simulink model "SkidSteeringControl"  (Simulink 8.9)
settings: Solver=VariableStepAuto  StartTime=0.0  StopTime=100  MaxStep=0.01  RelTol=1e-3
PreLoadFcn:
  | % Vehicle parameters
  | m = 1000;  % Vehicle mass
  | fR = 0.3;  % Front wheel radius
  | rR = 0.3;  % Rear wheel radius
  | J_front = 0.5;  % Front wheel moment of inertia
  | J_rear = 0.5;  % Rear wheel moment of inertia
  | J_engine = 0.01; % Engine moment of inertia
  | trans_ratio = 2.0;  % Transmission gear ratio
  | drive_ratio = 2.0;  % Final drive gear ratio
  | h = 0.5;   % Vehicle CG height above ground
  | 
  | % Aerodynamic load
  | cw = 0.34;  % Drag coefficient
  | rho = 1.18; % Air density
  | A_f = 1;    % Frontal area
  | 
  | 
  | %tire parameters
  | radiusWheel = 16*2.54/100;
  | inertiaLateral = 25*(radiusWheel)^2;
  | tireStiffness = 200000;
  | tireDamping = 1000;
StopFcn:
  | %%
  | close all;
  | figure;plot(disp_x,disp_y);grid on;axis('tight');
  | title('Vehicle Displacement Plot');
  | xlabel('Displacement X(m)');ylabel('Displacement Y(m)');
  | %%
  | figure;
  | subplot(2,1,1);
  | plot(desired_speedFL.time, desired_speedFL.signals.values,'g');grid on;hold on;
  | plot(desired_speedFR.time, desired_speedFR.signals.values,'b');grid on;
  | title('Desired Wheel Speed');
  | legend('Wheel Speed FL','Wheel Speed FR');
  | subplot(2,1,2);
  | plot(ref_speedFL.time, ref_speedFL.signals.values,'g');grid on;hold on;
  | plot(ref_speedFR.time, ref_speedFR.signals.values,'b');grid on;
  | title('Reference Wheel Speed(Slip Compensated)');
  | legend('Wheel Speed FL','Wheel Speed FR');
  | %%
  | figure;plot(yaw_rate.time,yaw_rate.signals.values);grid on;
  | title('Vehicle Yaw Rate');
  | xlabel('time(s)');ylabel('Yaw Rate(rad/s)');
  | %%
  | figure;
  | subplot(2,1,1);
  | plot(slip_WheelFL.time, slip_WheelFL.signals.values);grid on;
  | title('Wheel Slip Front Left');
  | xlabel('time(s)');ylabel('Slip Ratio');
  | subplot(2,1,2);
  | plot(slip_WheelFR.time, slip_WheelFR.signals.values);grid on;
  | title('Wheel Slip Front Right');
  | xlabel('time(s)');ylabel('Slip Ratio');
  | %%
  | figure;
  | subplot(2,1,1);
  | plot(torque_WheelFL.time, torque_WheelFL.signals.values);grid on;
  | title('Wheel Torque Front Left');
  | xlabel('time(s)');ylabel('Torque(Nm)');
  | subplot(2,1,2);
  | plot(torque_WheelFR.time, torque_WheelFR.signals.values);grid on;
  | title('Wheel Torque Front Right');
  | xlabel('time(s)');ylabel('Torque(Nm)');
libraries: nesl_utility x8, fl_lib x4, sdl_lib x4, simulink_extras x2, simulink x1
(part 1 of 2)
settings Model: Creator=divye  LastModifiedBy=divye
settings DataIOCC: LimitDataPoints=off  SaveFormat=Dataset  SignalLoggingSaveFormat=Dataset
settings OptimizationCC: LifeSpan=auto
settings DebuggingCC: UnderspecifiedInitializationDetection=Simplified  MergeDetectMultiDrivingBlocksExec=error  FcnCallInpInsideContextMsg=error  StateNameClashWarn=none  SFUnexpectedBacktrackingDiag=error  SFNoUnconditionalDefaultTransitionDiag=error  SFExecutionAtInitializationDiag=warning
settings HardwareCC: ProdBitPerPointer=64  ProdBitPerSizeT=64  ProdBitPerPtrDiffT=64  ProdLargestAtomicFloat=Float  ProdIntDivRoundTo=Zero  ProdEndianess=LittleEndian  ProdWordSize=64  ProdHWDeviceType=Intel->x86-64 (Windows64)
settings ModelReferenceCC: PropagateSignalLabelsOutOfModel=on
settings GRTTargetCC: TargetLangStandard=C99 (ISO)  GeneratePreprocessorConditionals=Use local settings  CombineOutputUpdateFcns=on  GRTInterface=off
settings ConfigComp: CovMetricSettings=dwe  CovHtmlReporting=off  CovSaveCumulativeToWorkspaceVar=off  CovSaveSingleToWorkspaceVar=off  CovExternalEMLEnable=on

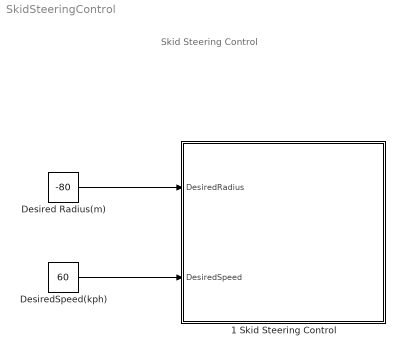
== system SkidSteeringControl ==
  note: Skid Steering Control
  1 Skid Steering Control : Subsystem
  Desired Radius(m) : Constant  Value=-80
  DesiredSpeed(kph) : Constant  Value=60
  wires:
  Desired Radius(m)/1 -> 1 Skid Steering Control/1(DesiredRadius)
  DesiredSpeed(kph)/1 -> 1 Skid Steering Control/2(DesiredSpeed)

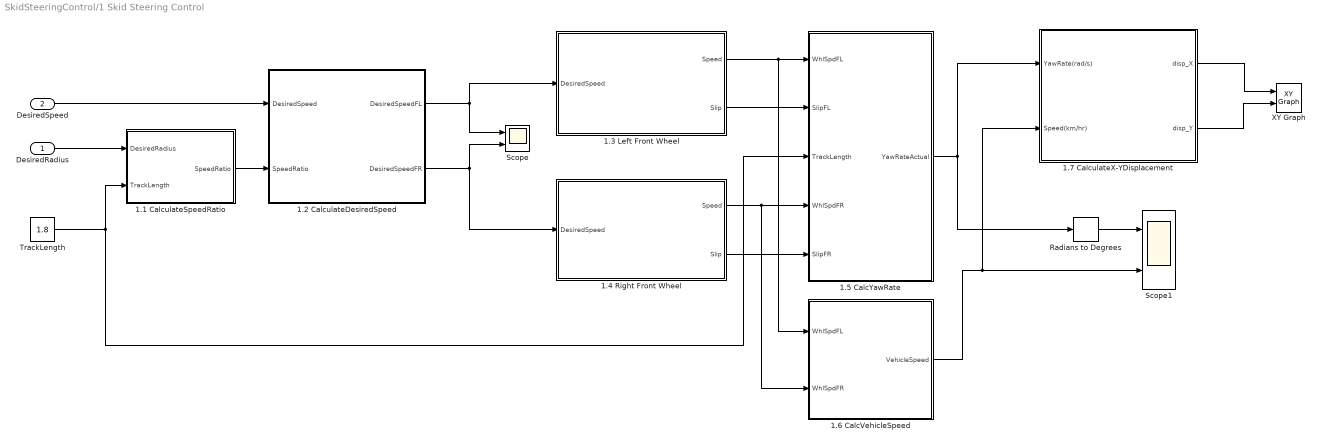
== system SkidSteeringControl/1 Skid Steering Control ==
  DesiredRadius : Inport
  DesiredSpeed : Inport  Port=2
  1.1 CalculateSpeedRatio : Subsystem
  1.2 CalculateDesiredSpeed : Subsystem
  1.3 Left Front Wheel : Subsystem
  1.4 Right Front Wheel : Subsystem
  1.5 CalcYawRate : Subsystem
  1.6 CalcVehicleSpeed : Subsystem
  1.7 CalculateX-YDisplacement : Subsystem
  Radians to Degrees : simulink_extras/Transformations/Radians to Degrees
  Scope : Scope  NumInputPorts=2
  Scope1 : Scope  NumInputPorts=2
  TrackLength : Constant  Value=1.8
  XY Graph : simulink/Sinks/XY Graph  xmin=-200  xmax=200  ymin=-200  ymax=200  st=-1
  wires:
  1.3 Left Front Wheel/1(Speed) -> 1.5 CalcYawRate/1(WhlSpdFL), 1.6 CalcVehicleSpeed/1(WhlSpdFL)
  TrackLength/1 -> 1.5 CalcYawRate/3(TrackLength), 1.1 CalculateSpeedRatio/2(TrackLength)
  1.5 CalcYawRate/1(YawRateActual) -> Radians to Degrees/1, 1.7 CalculateX-YDisplacement/1(YawRate(rad/s))
  1.6 CalcVehicleSpeed/1(VehicleSpeed) -> Scope1/2, 1.7 CalculateX-YDisplacement/2(Speed(km/hr))
  1.4 Right Front Wheel/1(Speed) -> 1.5 CalcYawRate/4(WhlSpdFR), 1.6 CalcVehicleSpeed/2(WhlSpdFR)
  1.4 Right Front Wheel/2(Slip) -> 1.5 CalcYawRate/5(SlipFR)
  1.3 Left Front Wheel/2(Slip) -> 1.5 CalcYawRate/2(SlipFL)
  DesiredSpeed/1 -> 1.2 CalculateDesiredSpeed/1(DesiredSpeed)
  Radians to Degrees/1 -> Scope1/1
  1.7 CalculateX-YDisplacement/1(disp_X) -> XY Graph/1
  1.7 CalculateX-YDisplacement/2(disp_Y) -> XY Graph/2
  1.2 CalculateDesiredSpeed/2(DesiredSpeedFR) -> 1.4 Right Front Wheel/1(DesiredSpeed), Scope/2
  1.2 CalculateDesiredSpeed/1(DesiredSpeedFL) -> Scope/1, 1.3 Left Front Wheel/1(DesiredSpeed)
  DesiredRadius/1 -> 1.1 CalculateSpeedRatio/1(DesiredRadius)
  1.1 CalculateSpeedRatio/1(SpeedRatio) -> 1.2 CalculateDesiredSpeed/2(SpeedRatio)

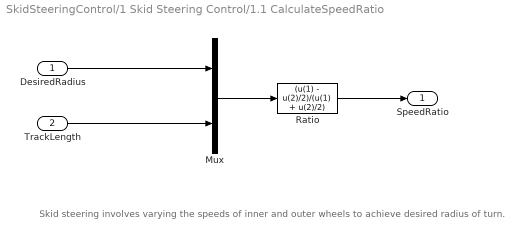
== system SkidSteeringControl/1 Skid Steering Control/1.1 CalculateSpeedRatio ==
  note: Skid steering involves varying the speeds of inner and outer wheels to achieve desired radius of turn.
  DesiredRadius : Inport
  TrackLength : Inport  Port=2
  Mux : Mux  Inputs=2
  Ratio : Fcn  Expr=(u(1) - u(2)/2)/(u(1) + u(2)/2)
  SpeedRatio : Outport
  wires:
  Ratio/1 -> SpeedRatio/1
  DesiredRadius/1 -> Mux/1
  Mux/1 -> Ratio/1
  TrackLength/1 -> Mux/2

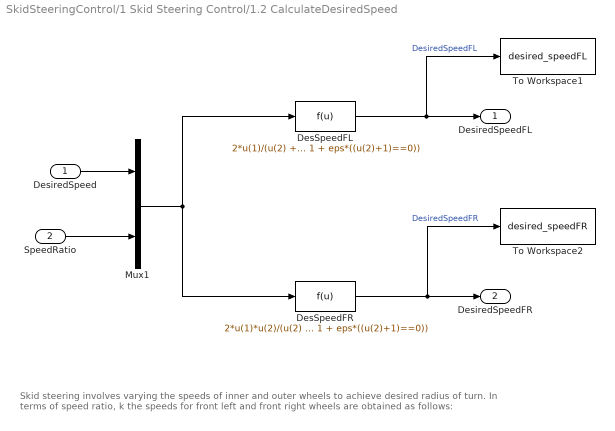
== system SkidSteeringControl/1 Skid Steering Control/1.2 CalculateDesiredSpeed ==
  note: Skid steering involves varying the speeds of inner and outer wheels to achieve desired radius of turn.
      |
      | In terms of speed ratio, k the speeds for front left and front right wheels are obtained as follows:
  DesiredSpeed : Inport
  SpeedRatio : Inport  Port=2
  DesSpeedFL : Fcn  Expr=2*u(1)/(u(2) + 1 + eps*((u(2)+1)==0))
  DesSpeedFR : Fcn  Expr=2*u(1)*u(2)/(u(2) + 1 + eps*((u(2)+1)==0))
  Mux1 : Mux  Inputs=2
  To Workspace1 : ToWorkspace  VariableName=desired_speedFL  SaveFormat=Structure With Time  SampleTime=-1
  To Workspace2 : ToWorkspace  VariableName=desired_speedFR  SaveFormat=Structure With Time  SampleTime=-1
  DesiredSpeedFL : Outport
  DesiredSpeedFR : Outport  Port=2
  wires:
  Mux1/1 -> DesSpeedFL/1, DesSpeedFR/1
  DesSpeedFR/1 -> To Workspace2/1, DesiredSpeedFR/1  "DesiredSpeedFR"
  DesSpeedFL/1 -> To Workspace1/1, DesiredSpeedFL/1  "DesiredSpeedFL"
  DesiredSpeed/1 -> Mux1/1
  SpeedRatio/1 -> Mux1/2

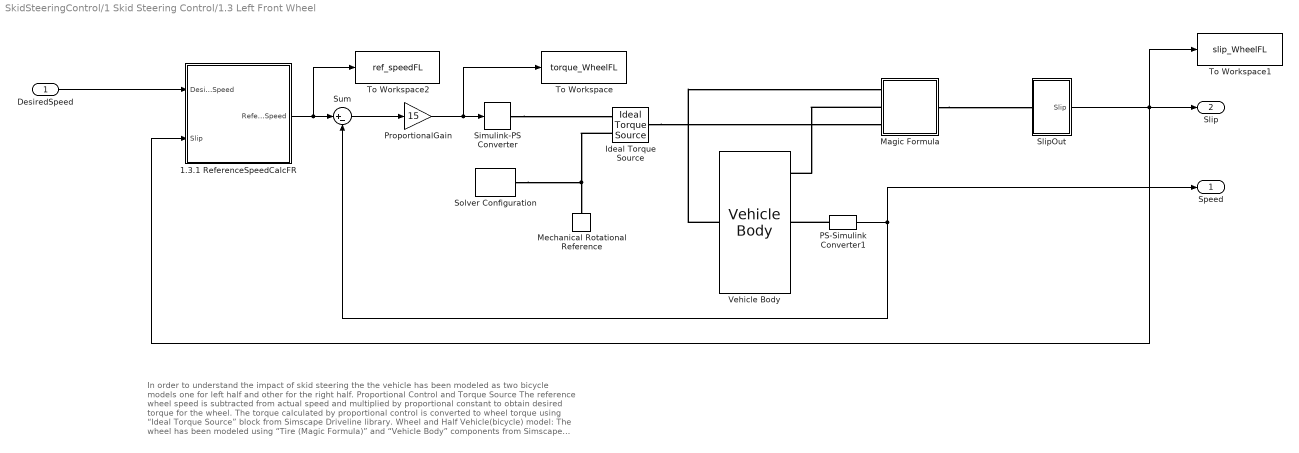
== system SkidSteeringControl/1 Skid Steering Control/1.3 Left Front Wheel ==
  note: In order to understand the impact of skid steering the the vehicle has been modeled as two bicycle models one for left half and other for the right half.
      | Proportional Control and Torque Source
      | The reference wheel speed is subtracted from actual speed and multiplied by proportional constant to obtain desired torque for the wheel.
      | The torque calculated by proportional control is converted to wheel torque using “Ideal Torque Source” block from Simscape Driveline library.
      | Wheel and Half Vehicle(bicycle) model:
      | The wheel has been modeled using “Tire (Magic Formula)” and “Vehicle Body” components from Simscape Driveline.
      | The Tire (Magic Formula) component requires Normal Force(N) and Wheel Torque(A).
      | Normal Force is provided as feedback from Vehicle Body component. In turn, the wheel component calculates slip ratio(S) and Hub Torque(H).
      | The vehicle body component takes the Hub Torque(H) calculated by Tire component and provides the Normal Force(N) and Speed(V).
  DesiredSpeed : Inport
  1.3.1 ReferenceSpeedCalcFR : Subsystem
  Ideal Torque Source : fl_lib/Mechanical/Mechanical Sources/Ideal Torque Source
  Magic Formula : Subsystem  VariantControl=MFormula
      mask Display:
      | plot([199.740630080105;207.645625381422;215.666495494822;223.725995056458;231.746506679781;239.614636200368], [285.533592122614;287.104128914395;287.892278108498;287.890449397339;287.098660392404;285.533592122614])
      | plot([182.29422131887;191.284049604609;200.547323621308;209.994832976365;219.535592990157;229.077720928241;238.529320882316;247.799368778054;256.798588986696;257.061044961602], [327.86290499758;331.09432156677;333.429020721321;334.844518032099;335.327181486212;334.872362770745;333.484442038558;331.176785725016;327.971617821912;327.86290499758])
      | plot([182.293066754937;199.741297401488], [327.862962149084;285.533680580556])
      | plot([239.613968878984;257.062199525535], [285.533680580556;327.862962149084])
      | plot([161.12998329239;162.078783791624;163.80431860203;166.28996988011;169.511799445263;173.438779317544;173.475674844307], [230.482414304504;238.453500201144;246.293204428793;253.926026350122;261.278457717503;268.279690597622;268.338450605791])
      | plot([115.521208412501;115.19363189143;115.795069625231;117.319729439748;119.752928027503;123.071232355974;127.242685340509;132.227113608518;137.976514391014;138.639091794056], [226.950718692202;236.412705455625;245.861238280392;255.205322630308;264.354969865087;273.222063880151;281.72120971289;289.770555942828;297.29258296555;298.068153121848])
      | plot([115.523664280772;161.128425970674], [226.952978409827;230.480418540537])
      | plot([173.474466428161;138.640995137393], [268.337409943342;298.068691045046])
      | plot([197.791294323752;190.505905487348;183.583957764389;177.092113295368;171.092892091325;165.644069931963;165.540704869119], [173.730032993176;177.080059057945;181.128046811489;185.835011918887;191.155623733067;197.038641853715;197.162104079289])
      | plot([187.018154556423;177.935574592276;169.151745387891;160.751260020237;152.815019755577;145.419454926048;138.635788863788;132.529351981303;127.158952603892;126.547993304079], [129.256249226993;131.857994736568;135.337460645285;139.661137794374;144.787386809327;150.666839109836;157.242872356214;164.45215575347;172.225259961496;173.223046112601])
      | plot([187.017316929996;197.78860732913], [129.25548478961;173.726426437497])
      | plot([165.537726134062;126.546914689243], [197.158707305789;173.222506418824])
      | plot([269.470357644972;273.38551933114;276.602305486856;279.089736702965;280.82385765709;281.787967816474;281.81616724833], [262.922159053497;255.989463868491;248.706398553292;241.143103008215;233.372415903877;225.469173204983;225.06588742066])
      | plot([304.431346528147;310.265227080294;315.332070863713;319.583081402952;322.977319142679;325.482095717982;327.073288761189;327.735574213461;327.462573903851;327.423015855416], [292.655530476138;285.116593543042;277.042138363134;268.509926353743;259.602127380701;250.404528417616;241.005707370423;231.496180023723;221.967528324303;221.475771485887])
      | plot([304.430681280792;269.471229985356], [292.651550844312;262.920269742608])
      | plot([281.817270442843;327.422032132745], [225.063278339803;221.472848206758])
      | plot([274.506490288884;269.03580586378;263.012187571475;256.493646148968;249.542958713556;242.227064184873;242.193171590222], [197.094155985096;191.184202827407;185.838928552521;181.109811073729;177.042394377551;173.675849910247;173.662235378073])
      | plot([313.374602600377;308.147922202874;302.181086731703;295.531560074253;288.263380807238;280.446545470191;272.156334460522;263.472587042146;254.478932449722;252.966160341391], [173.157457637183;165.349405231175;158.09125499764;151.452906891035;145.498291832517;140.284756020223;135.862508654033;132.274138393531;129.554203205929;129.189658564058])
      | plot([313.375261612236;274.510430172086], [173.15951641649;197.095717303455])
      | plot([242.196558974683;252.967849373817], [173.663436435163;129.192494787276])
      | plot([371.389053761959;370.658673461755;368.474566522701;364.857767088574;359.843106915069;353.478879920948;345.826377091206;336.959296211375;326.963032117569;315.933854297525;303.977979762811;291.210550120943;277.754522698759;263.739486396147;249.3004136741;234.576360696131;219.709128141403;204.841895586676;190.117842608706;175.678769886659;161.663733584047;148.207706161863;135.440276519995;123.484401985281;112.455224165237;102.458960071431;93.5918791916006;85.939376361858;79.5751493677372;74.5604891942319;70.9436897601051;68.7595828210511;68.0292025208473;68.7595828210511;70.9436897601053;74.5604891942321;79.5751493677375;85.9393763618583;93.5918791916009;102.458960071431;112.455224165237;123.484401985282;135.440276519995;148.207706161863;161.663733584048;175.67876988666;190.117842608707;204.841895586676;219.709128141403;234.576360696131;249.3004136741;263.739486396147;277.754522698759;291.210550120943;303.977979762811;315.933854297525;326.963032117569;336.959296211375;345.826377091205;353.478879920948;359.843106915069;364.857767088574;368.474566522701;370.658673461755;371.389053761959;371.389053761959;371.389053761959], [228.149788454175;213.282555899448;198.558502921478;184.119430199431;170.104393896819;156.648366474635;143.880936832767;131.925062298053;120.895884478009;110.899620384203;102.032539504372;94.3800366746299;88.0158096805091;83.0011495070038;79.3843500728769;77.2002431338229;76.4698628336191;77.2002431338229;79.3843500728769;83.0011495070038;88.0158096805092;94.38003667463;102.032539504373;110.899620384203;120.895884478009;131.925062298053;143.880936832767;156.648366474635;170.104393896819;184.119430199431;198.558502921479;213.282555899448;228.149788454175;243.017021008903;257.741073986872;272.180146708919;286.195183011531;299.651210433715;312.418640075584;324.374514610297;335.403692430341;345.399956524147;354.267037403978;361.91954023372;368.283767227841;373.298427401346;376.915226835473;379.099333774527;379.829714074731;379.099333774527;376.915226835473;373.298427401346;368.283767227841;361.91954023372;354.267037403978;345.399956524147;335.403692430341;324.374514610297;312.418640075583;299.651210433715;286.195183011531;272.180146708919;257.741073986872;243.017021008903;228.149788454176;228.149788454175;228.149788454175])
      | plot([363.45231346786;362.760150741504;360.690328467866;357.26278016692;352.510515002494;346.479299885972;339.227218715925;330.824112998412;321.350909235096;310.898839556798;299.568563108203;287.46919664527;274.717263681223;261.435572301422;247.752032454366;233.798424108965;219.709128141403;205.619832173842;191.666223828441;177.982683981384;164.700992601583;151.949059637537;139.849693174603;128.519416726008;118.067347047711;108.594143284395;100.191037566881;92.9389563968342;86.9077412803127;82.1554761158862;78.7279278149405;76.6581055413021;75.9659428149462;76.6581055413021;78.7279278149406;82.1554761158864;86.907741280313;92.9389563968345;100.191037566881;108.594143284395;118.067347047711;128.519416726009;139.849693174604;151.949059637537;164.700992601584;177.982683981384;191.666223828441;205.619832173842;219.709128141403;233.798424108965;247.752032454366;261.435572301422;274.717263681223;287.46919664527;299.568563108203;310.898839556798;321.350909235095;330.824112998411;339.227218715925;346.479299885972;352.510515002493;357.26278016692;360.690328467866;362.760150741504;363.45231346786;363.45231346786;363.45231346786], [228.149788454175;214.060492486614;200.106884141213;186.423344294156;173.141652914355;160.389719950309;148.290353487375;136.96007703878;126.508007360483;117.034803597167;108.631697879653;101.379616709606;95.3484015930846;90.596136428658;87.1685881277123;85.0987658540739;84.406603127718;85.0987658540739;87.1685881277124;90.5961364286582;95.3484015930846;101.379616709606;108.631697879653;117.034803597167;126.508007360483;136.960077038781;148.290353487376;160.389719950309;173.141652914355;186.423344294156;200.106884141213;214.060492486614;228.149788454175;242.239084421737;256.192692767138;269.876232614194;283.157923993995;295.909856958042;308.009223420975;319.33949986957;329.791569547868;339.264773311184;347.667879028697;354.919960198744;360.951175315265;365.703440479692;369.130988780638;371.200811054276;371.892973780632;371.200811054276;369.130988780638;365.703440479692;360.951175315265;354.919960198744;347.667879028697;339.264773311184;329.791569547868;319.33949986957;308.009223420975;295.909856958042;283.157923993995;269.876232614194;256.192692767138;242.239084421737;228.149788454176;228.149788454175;228.149788454175])
      | plot([261.408509686589;261.209838965396;260.615740109466;259.631934615548;258.267897068353;256.536763895118;254.455206854636;252.043272479101;249.324189015046;246.324142722634;243.072025687652;239.599157574934;235.93898400287;232.126754443812;228.199182752392;224.194093591025;220.150058157742;216.106022724459;212.100933563092;208.173361871672;204.361132312614;200.70095874055;197.228090627832;193.97597359285;190.975927300438;188.256843836383;185.844909460848;183.763352420366;182.032219247131;180.668181699936;179.684376206018;179.090277350088;178.891606628895;179.090277350088;179.684376206019;180.668181699936;182.032219247131;183.763352420366;185.844909460848;188.256843836383;190.975927300438;193.97597359285;197.228090627833;200.70095874055;204.361132312614;208.173361871672;212.100933563092;216.106022724459;220.150058157742;224.194093591025;228.199182752392;232.126754443812;235.93898400287;239.599157574934;243.072025687652;246.324142722634;249.324189015046;252.043272479101;254.455206854636;256.536763895118;258.267897068353;259.631934615548;260.615740109465;261.209838965396;261.408509686589;261.408509686589], [229.220618493855;225.176583060572;221.171493899205;217.243922207785;213.431692648727;209.771519076663;206.298650963945;203.046533928963;200.046487636551;197.327404172496;194.915469796961;192.833912756479;191.102779583244;189.738742036049;188.754936542131;188.160837686201;187.962166965008;188.160837686201;188.754936542131;189.738742036049;191.102779583244;192.833912756479;194.915469796961;197.327404172496;200.046487636551;203.046533928963;206.298650963945;209.771519076663;213.431692648727;217.243922207785;221.171493899205;225.176583060572;229.220618493855;233.264653927138;237.269743088505;241.197314779925;245.009544338983;248.669717911047;252.142586023765;255.394703058747;258.394749351159;261.113832815214;263.525767190749;265.607324231231;267.338457404466;268.702494951661;269.686300445579;270.280399301509;270.479070022702;270.280399301509;269.686300445579;268.702494951661;267.338457404466;265.607324231231;263.525767190749;261.113832815214;258.394749351159;255.394703058747;252.142586023765;248.669717911047;245.009544338983;241.197314779925;237.269743088505;233.264653927139;229.220618493855;229.220618493855])
      | plot([240.243868902326;240.144988512846;239.849299616612;239.359649859334;238.680754835845;237.819152676342;236.783141080621;235.58269740669;234.229382583359;232.736229772174;231.117618850946;229.38913792767;227.56743321852;225.670048735692;223.715257328969;221.721884708198;219.709128141403;217.696371574609;215.702998953837;213.748207547115;211.850823064286;210.029118355137;208.30063743186;206.682026510633;205.188873699447;203.835558876116;202.635115202186;201.599103606465;200.737501446962;200.058606423472;199.568956666194;199.27326776996;199.174387380481;199.27326776996;199.568956666194;200.058606423472;200.737501446962;201.599103606465;202.635115202186;203.835558876116;205.188873699447;206.682026510633;208.30063743186;210.029118355137;211.850823064286;213.748207547115;215.702998953837;217.696371574609;219.709128141403;221.721884708198;223.715257328969;225.670048735692;227.56743321852;229.38913792767;231.117618850946;232.736229772174;234.229382583359;235.58269740669;236.783141080621;237.819152676342;238.680754835845;239.359649859334;239.849299616612;240.144988512846;240.243868902326;240.243868902326], [230.66938854754;228.656631980745;226.663259359974;224.708467953251;222.811083470423;220.989378761273;219.260897837997;217.642286916769;216.149134105584;214.795819282253;213.595375608322;212.559364012601;211.697761853098;211.018866829609;210.529217072331;210.233528176097;210.134647786617;210.233528176097;210.529217072331;211.018866829609;211.697761853098;212.559364012601;213.595375608322;214.795819282253;216.149134105584;217.642286916769;219.260897837997;220.989378761273;222.811083470423;224.708467953251;226.663259359974;228.656631980745;230.66938854754;232.682145114334;234.675517735106;236.630309141828;238.527693624657;240.349398333806;242.077879257083;243.69649017831;245.189642989496;246.542957812827;247.743401486757;248.779413082478;249.641015241981;250.319910265471;250.809560022749;251.105248918983;251.204129308462;251.105248918983;250.809560022749;250.319910265471;249.641015241981;248.779413082478;247.743401486757;246.542957812827;245.189642989496;243.69649017831;242.077879257083;240.349398333806;238.527693624657;236.630309141828;234.675517735106;232.682145114334;230.66938854754;230.66938854754])
      | plot([339.327142573893;338.751149139472;337.02871596785;334.17643103205;330.22176339522;325.202798668544;319.167872225986;312.175103708213;304.291837298687;295.593993162365;286.165336293004;276.096669810484;265.484960477125;254.432404854758;243.045445095968;231.433743847976;219.709128141403;207.98451243483;196.372811186839;184.985851428048;173.933295805681;163.321586472322;153.252919989803;143.824263120442;135.126418984119;127.243152574594;120.250384056821;114.215457614262;109.196492887586;105.241825250756;102.389540314956;100.667107143335;100.091113708913;100.667107143335;102.389540314956;105.241825250756;109.196492887586;114.215457614262;120.250384056821;127.243152574594;135.12641898412;143.824263120442;153.252919989803;163.321586472323;173.933295805681;184.985851428048;196.372811186839;207.984512434831;219.709128141403;231.433743847976;243.045445095968;254.432404854758;265.484960477125;276.096669810484;286.165336293004;295.593993162365;304.291837298687;312.175103708212;319.167872225986;325.202798668544;330.22176339522;334.17643103205;337.02871596785;338.751149139472;339.327142573893;339.327142573893;339.327142573893], [228.149788454175;216.425172747602;204.813471499611;193.42651174082;182.373956118453;171.762246785094;161.693580302574;152.264923433213;143.567079296891;135.683812887366;128.691044369592;122.656117927034;117.637153200358;113.682485563528;110.830200627728;109.107767456107;108.531774021685;109.107767456107;110.830200627728;113.682485563528;117.637153200358;122.656117927034;128.691044369592;135.683812887366;143.567079296891;152.264923433214;161.693580302575;171.762246785094;182.373956118453;193.42651174082;204.813471499611;216.425172747602;228.149788454175;239.874404160748;251.48610540874;262.87306516753;273.925620789897;284.537330123256;294.605996605776;304.034653475137;312.732497611459;320.615764020985;327.608532538758;333.643458981316;338.662423707992;342.617091344822;345.469376280622;347.191809452243;347.767802886665;347.191809452243;345.469376280622;342.617091344822;338.662423707992;333.643458981316;327.608532538758;320.615764020985;312.732497611459;304.034653475137;294.605996605776;284.537330123256;273.925620789897;262.87306516753;251.48610540874;239.874404160748;228.149788454176;228.149788454175;228.149788454175])
      | plot([-20;467.858916595578;467.858916595578;-20;-20], [473.528016805649;473.528016805649;-20;-20;473.528016805649])
  Mechanical Rotational Reference : fl_lib/Mechanical/Rotational Elements/Mechanical Rotational Reference
  PS-Simulink Converter1 : nesl_utility/PS-Simulink Converter  PhysicalDomain=network_engine_domain  SubClassName=ps_output  LeftPortType=input  RightPortType=output  PseudoPeriodic=off  Frequencies=[]  Unit=km/hr  AffineConversion=off
  ProportionalGain : Gain  Gain=15
  Simulink-PS Converter : nesl_utility/Simulink-PS Converter  PhysicalDomain=network_engine_domain  SubClassName=ps_input  LeftPortType=input  RightPortType=output  PseudoPeriodic=off  Frequencies=[]  NoiseDistribution=none  NoiseParameters=[]  Unit=N*m  AffineConversion=off  FilteringAndDerivatives=provide  SimscapeFilterOrder=1  InputFilterTimeConstant=0.001  UdotUserProvided=0
  SlipOut : Subsystem
  Solver Configuration : nesl_utility/Solver Configuration  PhysicalDomain=network_engine_domain  SubClassName=solver  LeftPortType=input  RightPortType=generic  Accelerate=off  Tones=[]  Harmonics=[]  SimulateNoise=off  Profile=off  UseLocalSampling=off  EnableSwitchedLinearOptims=on  FrequencyDomain=off  UseCCode=off  RelTol=0.001  AbsTol=1e-06  MinStep=1e-09  ToWorkspace=off  RevertToSquareIcSolve=off  NumHomotopyIterations=100  PhasorMode=off  PhasorModeNumHarmonics=1  OverrideAbsTol=off  DoDC=off  ResidualTolerance=1e-9  UseLocalSolver=off  LocalSolverChoice=NE_BACKWARD_EULER_ADVANCER  LocalSolverSampleTime=0.001  DoFixedCost=off  MaxNonlinIter=3  MaxModeIter=2  LinearAlgebra=Sparse  DelaysMemoryBudget=1024  AutomaticFiltering=on  FilteringTimeConstant=0.001
  Sum : Sum  Inputs=|+-
  To Workspace : ToWorkspace  VariableName=torque_WheelFL  SaveFormat=Structure With Time  SampleTime=-1
  To Workspace1 : ToWorkspace  VariableName=slip_WheelFL  SaveFormat=Structure With Time  SampleTime=-1
  To Workspace2 : ToWorkspace  VariableName=ref_speedFL  SaveFormat=Structure With Time  SampleTime=-1
  Vehicle Body : sdl_lib/Tires & Vehicles/Vehicle Body  mass=1200 kg  n_w=2/2  x_f=1.4 m  x_r=1.6 m  y_c=0.5 m  area=3/2 m^2  Cd=0.4  g=9.81 m/s^2  rho=1.18 kg/m^3  v_specify=on  v_priority=High  v=0 m/s  v_nominal_specify=off  v_nominal_unit=m/s  v_nominal_value=1
      settings: SourceProductName=Simscape Driveline
  Speed : Outport
  Slip : Outport  Port=2
  wires:
  Sum/1 -> ProportionalGain/1
  1.3.1 ReferenceSpeedCalcFR/1(ReferenceSpeed) -> To Workspace2/1, Sum/1
  DesiredSpeed/1 -> 1.3.1 ReferenceSpeedCalcFR/1(DesiredSpeed)
  PS-Simulink Converter1/1 -> Speed/1, Sum/2
  ProportionalGain/1 -> To Workspace/1, Simulink-PS Converter/1
  SlipOut/1(Slip) -> To Workspace1/1, Slip/1, 1.3.1 ReferenceSpeedCalcFR/2("Slip ")
  connections:
  Vehicle Body/RConn2 -- Magic Formula/LConn1
  Ideal Torque Source/RConn2 -- Mechanical Rotational Reference/LConn1 -- Solver Configuration/RConn1
  Simulink-PS Converter/RConn1 -- Ideal Torque Source/RConn1
  PS-Simulink Converter1/LConn1 -- Vehicle Body/LConn2
  Magic Formula/RConn1 -- SlipOut/LConn1
  Magic Formula/LConn2 -- Vehicle Body/LConn1
  Ideal Torque Source/LConn1 -- Magic Formula/LConn3

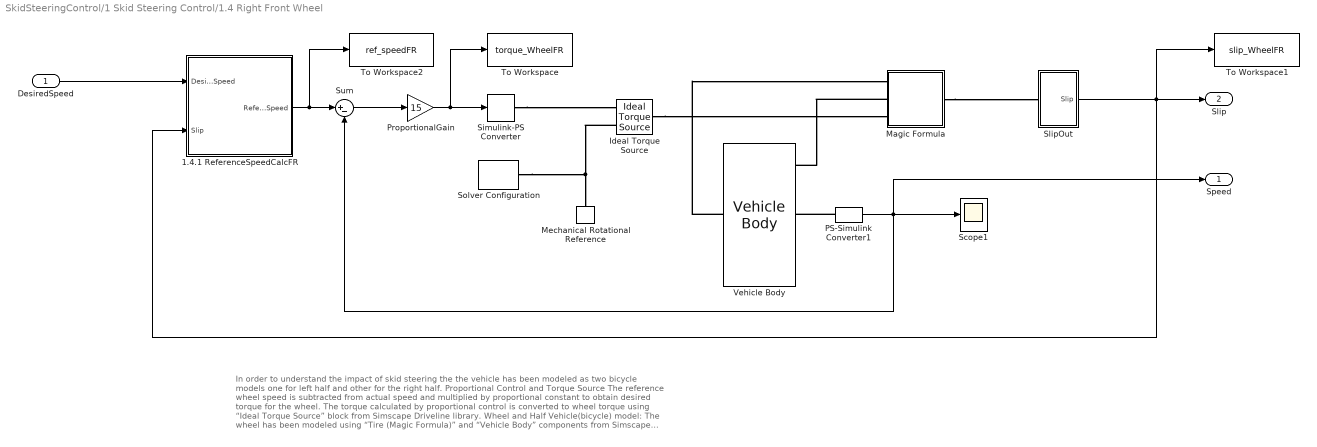
== system SkidSteeringControl/1 Skid Steering Control/1.4 Right Front Wheel ==
  note: In order to understand the impact of skid steering the the vehicle has been modeled as two bicycle models one for left half and other for the right half.
      | Proportional Control and Torque Source
      | The reference wheel speed is subtracted from actual speed and multiplied by proportional constant to obtain desired torque for the wheel.
      | The torque calculated by proportional control is converted to wheel torque using “Ideal Torque Source” block from Simscape Driveline library.
      | Wheel and Half Vehicle(bicycle) model:
      | The wheel has been modeled using “Tire (Magic Formula)” and “Vehicle Body” components from Simscape Driveline.
      | The Tire (Magic Formula) component requires Normal Force(N) and Wheel Torque(A).
      | Normal Force is provided as feedback from Vehicle Body component. In turn, the wheel component calculates slip ratio(S) and Hub Torque(H).
      | The vehicle body component takes the Hub Torque(H) calculated by Tire component and provides the Normal Force(N) and Speed(V).
  DesiredSpeed : Inport
  1.4.1 ReferenceSpeedCalcFR : Subsystem
  Ideal Torque Source : fl_lib/Mechanical/Mechanical Sources/Ideal Torque Source
  Magic Formula : Subsystem  VariantControl=MFormula
      mask Display:
      | plot([199.740630080105;207.645625381422;215.666495494822;223.725995056458;231.746506679781;239.614636200368], [285.533592122614;287.104128914395;287.892278108498;287.890449397339;287.098660392404;285.533592122614])
      | plot([182.29422131887;191.284049604609;200.547323621308;209.994832976365;219.535592990157;229.077720928241;238.529320882316;247.799368778054;256.798588986696;257.061044961602], [327.86290499758;331.09432156677;333.429020721321;334.844518032099;335.327181486212;334.872362770745;333.484442038558;331.176785725016;327.971617821912;327.86290499758])
      | plot([182.293066754937;199.741297401488], [327.862962149084;285.533680580556])
      | plot([239.613968878984;257.062199525535], [285.533680580556;327.862962149084])
      | plot([161.12998329239;162.078783791624;163.80431860203;166.28996988011;169.511799445263;173.438779317544;173.475674844307], [230.482414304504;238.453500201144;246.293204428793;253.926026350122;261.278457717503;268.279690597622;268.338450605791])
      | plot([115.521208412501;115.19363189143;115.795069625231;117.319729439748;119.752928027503;123.071232355974;127.242685340509;132.227113608518;137.976514391014;138.639091794056], [226.950718692202;236.412705455625;245.861238280392;255.205322630308;264.354969865087;273.222063880151;281.72120971289;289.770555942828;297.29258296555;298.068153121848])
      | plot([115.523664280772;161.128425970674], [226.952978409827;230.480418540537])
      | plot([173.474466428161;138.640995137393], [268.337409943342;298.068691045046])
      | plot([197.791294323752;190.505905487348;183.583957764389;177.092113295368;171.092892091325;165.644069931963;165.540704869119], [173.730032993176;177.080059057945;181.128046811489;185.835011918887;191.155623733067;197.038641853715;197.162104079289])
      | plot([187.018154556423;177.935574592276;169.151745387891;160.751260020237;152.815019755577;145.419454926048;138.635788863788;132.529351981303;127.158952603892;126.547993304079], [129.256249226993;131.857994736568;135.337460645285;139.661137794374;144.787386809327;150.666839109836;157.242872356214;164.45215575347;172.225259961496;173.223046112601])
      | plot([187.017316929996;197.78860732913], [129.25548478961;173.726426437497])
      | plot([165.537726134062;126.546914689243], [197.158707305789;173.222506418824])
      | plot([269.470357644972;273.38551933114;276.602305486856;279.089736702965;280.82385765709;281.787967816474;281.81616724833], [262.922159053497;255.989463868491;248.706398553292;241.143103008215;233.372415903877;225.469173204983;225.06588742066])
      | plot([304.431346528147;310.265227080294;315.332070863713;319.583081402952;322.977319142679;325.482095717982;327.073288761189;327.735574213461;327.462573903851;327.423015855416], [292.655530476138;285.116593543042;277.042138363134;268.509926353743;259.602127380701;250.404528417616;241.005707370423;231.496180023723;221.967528324303;221.475771485887])
      | plot([304.430681280792;269.471229985356], [292.651550844312;262.920269742608])
      | plot([281.817270442843;327.422032132745], [225.063278339803;221.472848206758])
      | plot([274.506490288884;269.03580586378;263.012187571475;256.493646148968;249.542958713556;242.227064184873;242.193171590222], [197.094155985096;191.184202827407;185.838928552521;181.109811073729;177.042394377551;173.675849910247;173.662235378073])
      | plot([313.374602600377;308.147922202874;302.181086731703;295.531560074253;288.263380807238;280.446545470191;272.156334460522;263.472587042146;254.478932449722;252.966160341391], [173.157457637183;165.349405231175;158.09125499764;151.452906891035;145.498291832517;140.284756020223;135.862508654033;132.274138393531;129.554203205929;129.189658564058])
      | plot([313.375261612236;274.510430172086], [173.15951641649;197.095717303455])
      | plot([242.196558974683;252.967849373817], [173.663436435163;129.192494787276])
      | plot([371.389053761959;370.658673461755;368.474566522701;364.857767088574;359.843106915069;353.478879920948;345.826377091206;336.959296211375;326.963032117569;315.933854297525;303.977979762811;291.210550120943;277.754522698759;263.739486396147;249.3004136741;234.576360696131;219.709128141403;204.841895586676;190.117842608706;175.678769886659;161.663733584047;148.207706161863;135.440276519995;123.484401985281;112.455224165237;102.458960071431;93.5918791916006;85.939376361858;79.5751493677372;74.5604891942319;70.9436897601051;68.7595828210511;68.0292025208473;68.7595828210511;70.9436897601053;74.5604891942321;79.5751493677375;85.9393763618583;93.5918791916009;102.458960071431;112.455224165237;123.484401985282;135.440276519995;148.207706161863;161.663733584048;175.67876988666;190.117842608707;204.841895586676;219.709128141403;234.576360696131;249.3004136741;263.739486396147;277.754522698759;291.210550120943;303.977979762811;315.933854297525;326.963032117569;336.959296211375;345.826377091205;353.478879920948;359.843106915069;364.857767088574;368.474566522701;370.658673461755;371.389053761959;371.389053761959;371.389053761959], [228.149788454175;213.282555899448;198.558502921478;184.119430199431;170.104393896819;156.648366474635;143.880936832767;131.925062298053;120.895884478009;110.899620384203;102.032539504372;94.3800366746299;88.0158096805091;83.0011495070038;79.3843500728769;77.2002431338229;76.4698628336191;77.2002431338229;79.3843500728769;83.0011495070038;88.0158096805092;94.38003667463;102.032539504373;110.899620384203;120.895884478009;131.925062298053;143.880936832767;156.648366474635;170.104393896819;184.119430199431;198.558502921479;213.282555899448;228.149788454175;243.017021008903;257.741073986872;272.180146708919;286.195183011531;299.651210433715;312.418640075584;324.374514610297;335.403692430341;345.399956524147;354.267037403978;361.91954023372;368.283767227841;373.298427401346;376.915226835473;379.099333774527;379.829714074731;379.099333774527;376.915226835473;373.298427401346;368.283767227841;361.91954023372;354.267037403978;345.399956524147;335.403692430341;324.374514610297;312.418640075583;299.651210433715;286.195183011531;272.180146708919;257.741073986872;243.017021008903;228.149788454176;228.149788454175;228.149788454175])
      | plot([363.45231346786;362.760150741504;360.690328467866;357.26278016692;352.510515002494;346.479299885972;339.227218715925;330.824112998412;321.350909235096;310.898839556798;299.568563108203;287.46919664527;274.717263681223;261.435572301422;247.752032454366;233.798424108965;219.709128141403;205.619832173842;191.666223828441;177.982683981384;164.700992601583;151.949059637537;139.849693174603;128.519416726008;118.067347047711;108.594143284395;100.191037566881;92.9389563968342;86.9077412803127;82.1554761158862;78.7279278149405;76.6581055413021;75.9659428149462;76.6581055413021;78.7279278149406;82.1554761158864;86.907741280313;92.9389563968345;100.191037566881;108.594143284395;118.067347047711;128.519416726009;139.849693174604;151.949059637537;164.700992601584;177.982683981384;191.666223828441;205.619832173842;219.709128141403;233.798424108965;247.752032454366;261.435572301422;274.717263681223;287.46919664527;299.568563108203;310.898839556798;321.350909235095;330.824112998411;339.227218715925;346.479299885972;352.510515002493;357.26278016692;360.690328467866;362.760150741504;363.45231346786;363.45231346786;363.45231346786], [228.149788454175;214.060492486614;200.106884141213;186.423344294156;173.141652914355;160.389719950309;148.290353487375;136.96007703878;126.508007360483;117.034803597167;108.631697879653;101.379616709606;95.3484015930846;90.596136428658;87.1685881277123;85.0987658540739;84.406603127718;85.0987658540739;87.1685881277124;90.5961364286582;95.3484015930846;101.379616709606;108.631697879653;117.034803597167;126.508007360483;136.960077038781;148.290353487376;160.389719950309;173.141652914355;186.423344294156;200.106884141213;214.060492486614;228.149788454175;242.239084421737;256.192692767138;269.876232614194;283.157923993995;295.909856958042;308.009223420975;319.33949986957;329.791569547868;339.264773311184;347.667879028697;354.919960198744;360.951175315265;365.703440479692;369.130988780638;371.200811054276;371.892973780632;371.200811054276;369.130988780638;365.703440479692;360.951175315265;354.919960198744;347.667879028697;339.264773311184;329.791569547868;319.33949986957;308.009223420975;295.909856958042;283.157923993995;269.876232614194;256.192692767138;242.239084421737;228.149788454176;228.149788454175;228.149788454175])
      | plot([261.408509686589;261.209838965396;260.615740109466;259.631934615548;258.267897068353;256.536763895118;254.455206854636;252.043272479101;249.324189015046;246.324142722634;243.072025687652;239.599157574934;235.93898400287;232.126754443812;228.199182752392;224.194093591025;220.150058157742;216.106022724459;212.100933563092;208.173361871672;204.361132312614;200.70095874055;197.228090627832;193.97597359285;190.975927300438;188.256843836383;185.844909460848;183.763352420366;182.032219247131;180.668181699936;179.684376206018;179.090277350088;178.891606628895;179.090277350088;179.684376206019;180.668181699936;182.032219247131;183.763352420366;185.844909460848;188.256843836383;190.975927300438;193.97597359285;197.228090627833;200.70095874055;204.361132312614;208.173361871672;212.100933563092;216.106022724459;220.150058157742;224.194093591025;228.199182752392;232.126754443812;235.93898400287;239.599157574934;243.072025687652;246.324142722634;249.324189015046;252.043272479101;254.455206854636;256.536763895118;258.267897068353;259.631934615548;260.615740109465;261.209838965396;261.408509686589;261.408509686589], [229.220618493855;225.176583060572;221.171493899205;217.243922207785;213.431692648727;209.771519076663;206.298650963945;203.046533928963;200.046487636551;197.327404172496;194.915469796961;192.833912756479;191.102779583244;189.738742036049;188.754936542131;188.160837686201;187.962166965008;188.160837686201;188.754936542131;189.738742036049;191.102779583244;192.833912756479;194.915469796961;197.327404172496;200.046487636551;203.046533928963;206.298650963945;209.771519076663;213.431692648727;217.243922207785;221.171493899205;225.176583060572;229.220618493855;233.264653927138;237.269743088505;241.197314779925;245.009544338983;248.669717911047;252.142586023765;255.394703058747;258.394749351159;261.113832815214;263.525767190749;265.607324231231;267.338457404466;268.702494951661;269.686300445579;270.280399301509;270.479070022702;270.280399301509;269.686300445579;268.702494951661;267.338457404466;265.607324231231;263.525767190749;261.113832815214;258.394749351159;255.394703058747;252.142586023765;248.669717911047;245.009544338983;241.197314779925;237.269743088505;233.264653927139;229.220618493855;229.220618493855])
      | plot([240.243868902326;240.144988512846;239.849299616612;239.359649859334;238.680754835845;237.819152676342;236.783141080621;235.58269740669;234.229382583359;232.736229772174;231.117618850946;229.38913792767;227.56743321852;225.670048735692;223.715257328969;221.721884708198;219.709128141403;217.696371574609;215.702998953837;213.748207547115;211.850823064286;210.029118355137;208.30063743186;206.682026510633;205.188873699447;203.835558876116;202.635115202186;201.599103606465;200.737501446962;200.058606423472;199.568956666194;199.27326776996;199.174387380481;199.27326776996;199.568956666194;200.058606423472;200.737501446962;201.599103606465;202.635115202186;203.835558876116;205.188873699447;206.682026510633;208.30063743186;210.029118355137;211.850823064286;213.748207547115;215.702998953837;217.696371574609;219.709128141403;221.721884708198;223.715257328969;225.670048735692;227.56743321852;229.38913792767;231.117618850946;232.736229772174;234.229382583359;235.58269740669;236.783141080621;237.819152676342;238.680754835845;239.359649859334;239.849299616612;240.144988512846;240.243868902326;240.243868902326], [230.66938854754;228.656631980745;226.663259359974;224.708467953251;222.811083470423;220.989378761273;219.260897837997;217.642286916769;216.149134105584;214.795819282253;213.595375608322;212.559364012601;211.697761853098;211.018866829609;210.529217072331;210.233528176097;210.134647786617;210.233528176097;210.529217072331;211.018866829609;211.697761853098;212.559364012601;213.595375608322;214.795819282253;216.149134105584;217.642286916769;219.260897837997;220.989378761273;222.811083470423;224.708467953251;226.663259359974;228.656631980745;230.66938854754;232.682145114334;234.675517735106;236.630309141828;238.527693624657;240.349398333806;242.077879257083;243.69649017831;245.189642989496;246.542957812827;247.743401486757;248.779413082478;249.641015241981;250.319910265471;250.809560022749;251.105248918983;251.204129308462;251.105248918983;250.809560022749;250.319910265471;249.641015241981;248.779413082478;247.743401486757;246.542957812827;245.189642989496;243.69649017831;242.077879257083;240.349398333806;238.527693624657;236.630309141828;234.675517735106;232.682145114334;230.66938854754;230.66938854754])
      | plot([339.327142573893;338.751149139472;337.02871596785;334.17643103205;330.22176339522;325.202798668544;319.167872225986;312.175103708213;304.291837298687;295.593993162365;286.165336293004;276.096669810484;265.484960477125;254.432404854758;243.045445095968;231.433743847976;219.709128141403;207.98451243483;196.372811186839;184.985851428048;173.933295805681;163.321586472322;153.252919989803;143.824263120442;135.126418984119;127.243152574594;120.250384056821;114.215457614262;109.196492887586;105.241825250756;102.389540314956;100.667107143335;100.091113708913;100.667107143335;102.389540314956;105.241825250756;109.196492887586;114.215457614262;120.250384056821;127.243152574594;135.12641898412;143.824263120442;153.252919989803;163.321586472323;173.933295805681;184.985851428048;196.372811186839;207.984512434831;219.709128141403;231.433743847976;243.045445095968;254.432404854758;265.484960477125;276.096669810484;286.165336293004;295.593993162365;304.291837298687;312.175103708212;319.167872225986;325.202798668544;330.22176339522;334.17643103205;337.02871596785;338.751149139472;339.327142573893;339.327142573893;339.327142573893], [228.149788454175;216.425172747602;204.813471499611;193.42651174082;182.373956118453;171.762246785094;161.693580302574;152.264923433213;143.567079296891;135.683812887366;128.691044369592;122.656117927034;117.637153200358;113.682485563528;110.830200627728;109.107767456107;108.531774021685;109.107767456107;110.830200627728;113.682485563528;117.637153200358;122.656117927034;128.691044369592;135.683812887366;143.567079296891;152.264923433214;161.693580302575;171.762246785094;182.373956118453;193.42651174082;204.813471499611;216.425172747602;228.149788454175;239.874404160748;251.48610540874;262.87306516753;273.925620789897;284.537330123256;294.605996605776;304.034653475137;312.732497611459;320.615764020985;327.608532538758;333.643458981316;338.662423707992;342.617091344822;345.469376280622;347.191809452243;347.767802886665;347.191809452243;345.469376280622;342.617091344822;338.662423707992;333.643458981316;327.608532538758;320.615764020985;312.732497611459;304.034653475137;294.605996605776;284.537330123256;273.925620789897;262.87306516753;251.48610540874;239.874404160748;228.149788454176;228.149788454175;228.149788454175])
      | plot([-20;467.858916595578;467.858916595578;-20;-20], [473.528016805649;473.528016805649;-20;-20;473.528016805649])
  Mechanical Rotational Reference : fl_lib/Mechanical/Rotational Elements/Mechanical Rotational Reference
  PS-Simulink Converter1 : nesl_utility/PS-Simulink Converter  PhysicalDomain=network_engine_domain  SubClassName=ps_output  LeftPortType=input  RightPortType=output  PseudoPeriodic=off  Frequencies=[]  Unit=km/hr  AffineConversion=off
  ProportionalGain : Gain  Gain=15
  Scope1 : Scope
  Simulink-PS Converter : nesl_utility/Simulink-PS Converter  PhysicalDomain=network_engine_domain  SubClassName=ps_input  LeftPortType=input  RightPortType=output  PseudoPeriodic=off  Frequencies=[]  NoiseDistribution=none  NoiseParameters=[]  Unit=N*m  AffineConversion=off  FilteringAndDerivatives=provide  SimscapeFilterOrder=1  InputFilterTimeConstant=0.001  UdotUserProvided=0
  SlipOut : Subsystem
  Solver Configuration : nesl_utility/Solver Configuration  PhysicalDomain=network_engine_domain  SubClassName=solver  LeftPortType=input  RightPortType=generic  Accelerate=off  Tones=[]  Harmonics=[]  SimulateNoise=off  Profile=off  UseLocalSampling=off  EnableSwitchedLinearOptims=on  FrequencyDomain=off  UseCCode=off  RelTol=0.001  AbsTol=1e-06  MinStep=1e-09  ToWorkspace=off  RevertToSquareIcSolve=off  NumHomotopyIterations=100  PhasorMode=off  PhasorModeNumHarmonics=1  OverrideAbsTol=off  DoDC=off  ResidualTolerance=1e-9  UseLocalSolver=off  LocalSolverChoice=NE_BACKWARD_EULER_ADVANCER  LocalSolverSampleTime=0.001  DoFixedCost=off  MaxNonlinIter=3  MaxModeIter=2  LinearAlgebra=Sparse  DelaysMemoryBudget=1024  AutomaticFiltering=on  FilteringTimeConstant=0.001
  Sum : Sum  Inputs=|+-
  To Workspace : ToWorkspace  VariableName=torque_WheelFR  SaveFormat=Structure With Time  SampleTime=-1
  To Workspace1 : ToWorkspace  VariableName=slip_WheelFR  SaveFormat=Structure With Time  SampleTime=-1
  To Workspace2 : ToWorkspace  VariableName=ref_speedFR  SaveFormat=Structure With Time  SampleTime=-1
  Vehicle Body : sdl_lib/Tires & Vehicles/Vehicle Body  mass=1200 kg  n_w=2/2  x_f=1.4 m  x_r=1.6 m  y_c=0.5 m  area=3/2 m^2  Cd=0.4  g=9.81 m/s^2  rho=1.18 kg/m^3  v_specify=on  v_priority=High  v=0 m/s  v_nominal_specify=off  v_nominal_unit=m/s  v_nominal_value=1
      settings: SourceProductName=Simscape Driveline
  Speed : Outport
  Slip : Outport  Port=2
  wires:
  Sum/1 -> ProportionalGain/1
  1.4.1 ReferenceSpeedCalcFR/1(ReferenceSpeed) -> To Workspace2/1, Sum/1
  DesiredSpeed/1 -> 1.4.1 ReferenceSpeedCalcFR/1(DesiredSpeed)
  PS-Simulink Converter1/1 -> Speed/1, Scope1/1, Sum/2
  ProportionalGain/1 -> To Workspace/1, Simulink-PS Converter/1
  SlipOut/1(Slip) -> To Workspace1/1, Slip/1, 1.4.1 ReferenceSpeedCalcFR/2("Slip ")
  connections:
  Vehicle Body/RConn2 -- Magic Formula/LConn1
  Solver Configuration/RConn1 -- Ideal Torque Source/RConn2 -- Mechanical Rotational Reference/LConn1
  Simulink-PS Converter/RConn1 -- Ideal Torque Source/RConn1
  PS-Simulink Converter1/LConn1 -- Vehicle Body/LConn2
  Magic Formula/RConn1 -- SlipOut/LConn1
  Magic Formula/LConn2 -- Vehicle Body/LConn1
  Ideal Torque Source/LConn1 -- Magic Formula/LConn3

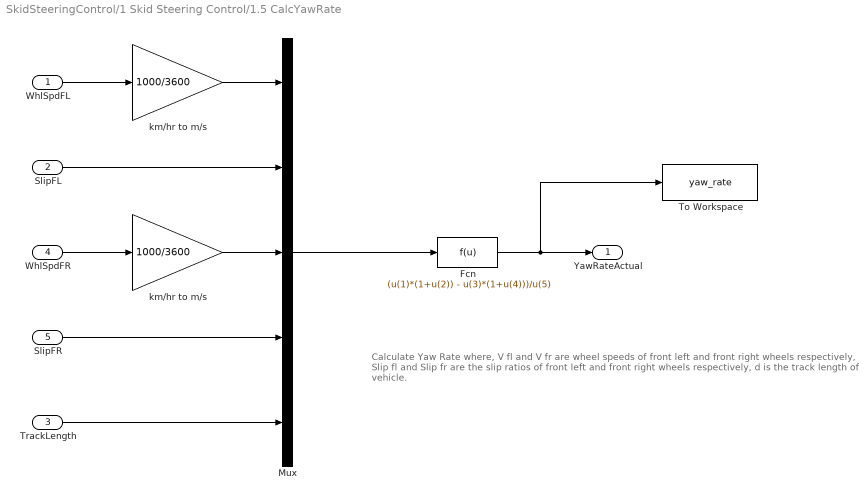
== system SkidSteeringControl/1 Skid Steering Control/1.5 CalcYawRate ==
  note: Calculate Yaw Rate
      |
      | where, V fl and V fr are wheel speeds of front left and front right wheels respectively,
      | Slip fl and Slip fr are the slip ratios of front left and front right wheels respectively, d is the track length of vehicle.
  WhlSpdFL : Inport
  SlipFL : Inport  Port=2
  TrackLength : Inport  Port=3
  WhlSpdFR : Inport  Port=4
  SlipFR : Inport  Port=5
  Fcn : Fcn  Expr=(u(1)*(1+u(2)) - u(3)*(1+u(4)))/u(5)
  Mux : Mux  Inputs=5
  To Workspace : ToWorkspace  VariableName=yaw_rate  SaveFormat=Structure With Time  SampleTime=-1
  km/hr to m/s : Gain  Gain=1000/3600
  "km/hr to m/s " : Gain  Gain=1000/3600
  YawRateActual : Outport
  wires:
  Fcn/1 -> To Workspace/1, YawRateActual/1
  WhlSpdFR/1 -> "km/hr to m/s "/1
  SlipFL/1 -> Mux/2
  WhlSpdFL/1 -> km/hr to m/s/1
  SlipFR/1 -> Mux/4
  TrackLength/1 -> Mux/5
  Mux/1 -> Fcn/1
  km/hr to m/s/1 -> Mux/1
  "km/hr to m/s "/1 -> Mux/3

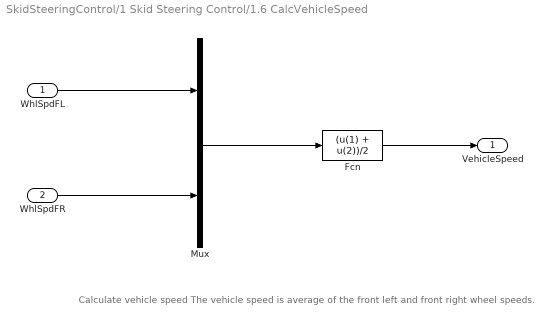
== system SkidSteeringControl/1 Skid Steering Control/1.6 CalcVehicleSpeed ==
  note: Calculate vehicle speed
      | The vehicle speed is average of the front left and front right wheel speeds.
  WhlSpdFL : Inport
  WhlSpdFR : Inport  Port=2
  Fcn : Fcn  Expr=(u(1) + u(2))/2
  Mux : Mux  Inputs=2
  VehicleSpeed : Outport
  wires:
  Fcn/1 -> VehicleSpeed/1
  WhlSpdFR/1 -> Mux/2
  WhlSpdFL/1 -> Mux/1
  Mux/1 -> Fcn/1

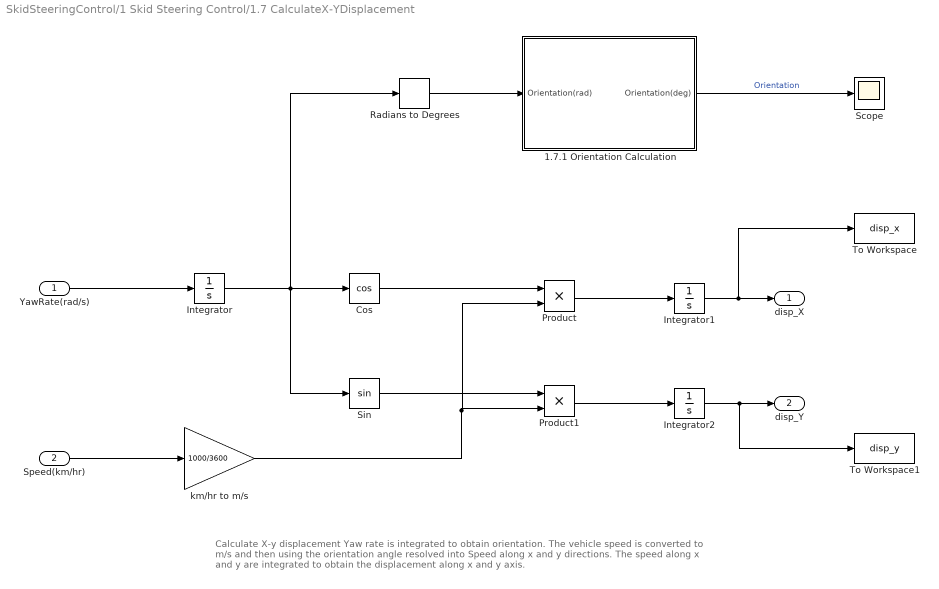
== system SkidSteeringControl/1 Skid Steering Control/1.7 CalculateX-YDisplacement ==
  note: Calculate X-y displacement
      | Yaw rate is integrated to obtain orientation.
      | The vehicle speed is converted to m/s and then using the orientation angle resolved into Speed along x and y directions.
      | The speed along x and y are integrated to obtain the displacement along x and y axis.
  YawRate(rad/s) : Inport
  Speed(km/hr) : Inport  Port=2
  1.7.1 Orientation Calculation : Subsystem
  Cos : Trigonometry  Operator=cos
  Integrator : Integrator
  Integrator1 : Integrator
  Integrator2 : Integrator
  Product : Product
  Product1 : Product
  Radians to Degrees : simulink_extras/Transformations/Radians to Degrees
  Scope : Scope
  Sin : Trigonometry
  To Workspace : ToWorkspace  VariableName=disp_x  SampleTime=-1
  To Workspace1 : ToWorkspace  VariableName=disp_y  SampleTime=-1
  km/hr to m/s : Gain  Gain=1000/3600
  disp_X : Outport
  disp_Y : Outport  Port=2
  wires:
  Speed(km/hr)/1 -> km/hr to m/s/1
  Sin/1 -> Product1/1
  Product/1 -> Integrator1/1
  Product1/1 -> Integrator2/1
  Integrator/1 -> Radians to Degrees/1, Sin/1, Cos/1
  YawRate(rad/s)/1 -> Integrator/1
  Cos/1 -> Product/1
  km/hr to m/s/1 -> Product/2, Product1/2
  Integrator1/1 -> To Workspace/1, disp_X/1
  Integrator2/1 -> To Workspace1/1, disp_Y/1
  1.7.1 Orientation Calculation/1(Orientation(deg)) -> Scope/1  "Orientation"
  Radians to Degrees/1 -> 1.7.1 Orientation Calculation/1(Orientation(rad))
